simulink model "aeb_sim"  (R2023b)
settings: Solver=ode3  StartTime=0.0  StopTime=t_end  FixedStep=Ts  RelTol=1e-3
values from neighbouring files (symbols this model uses):
  a_cmd_max = 9    [aeb_parameter.m]
  AEB_enable = true    [aeb_parameter.m]
  ax_emergency = 0.90*g    (= 8.829)    [aeb_parameter.m]
  ax_moderate = 0.70*g    (= 6.867)    [aeb_parameter.m]
  ax_partial = 0.45*g    (= 4.4145)    [aeb_parameter.m]
  bias_TTC = 0.05    [aeb_parameter.m]
  CdA = 0.65    [aeb_parameter.m]
  Crr = 0.020    (= 0.02)    [aeb_parameter.m]
  ego_v0 = 27.77    [aeb_parameter.m]
  ego_x0 = 0.0    (= 0)    [aeb_parameter.m]
  eps_v = 0.05    [aeb_parameter.m]
  g = 9.81    [aeb_parameter.m]
  jerk_lim = 20    [aeb_parameter.m]
  m = 2000    [aeb_parameter.m]
  mu = struct('dry',mu_dry,'wet',mu_wet,'ice',mu_ice).(mu_case)    [aeb_parameter.m]
  R_safe = 2.0    (= 2)    [aeb_parameter.m]
  rho_air = 1.2    [aeb_parameter.m]
  tau_brk = 0.08    [aeb_parameter.m]
  tgt_a = -4    [aeb_parameter.m]
  tgt_v0 = 20.83    [aeb_parameter.m]
  tgt_x0 = 45    [aeb_parameter.m]
  TTCbrk = 1.8    [aeb_parameter.m]
  TTCfull = 1.2    [aeb_parameter.m]
  TTClow = 2.6    [aeb_parameter.m]
settings Model: Creator=PRATIK  LastModifiedBy=PRATIK
settings DataIOCC: SaveState=on
settings OptimizationCC: UseDivisionForNetSlopeComputation=on

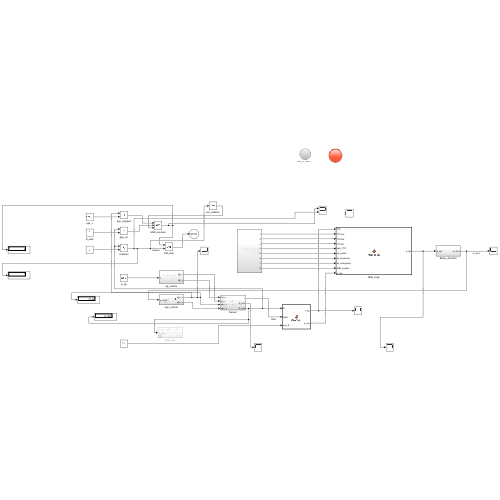
[thumbnail: Simulink's stored preview of the top-level diagram]
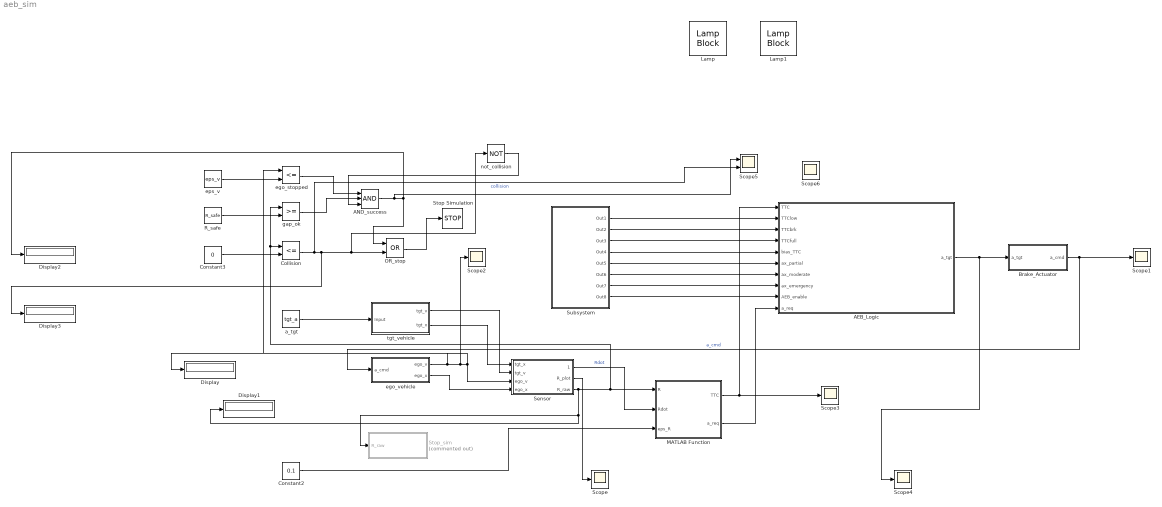
== system aeb_sim ==
  AEB_Logic : MATLAB Function  TreatAsAtomicUnit=on
  AND_success : Logic  Inputs=3  AllPortsSameDT=off  OutDataTypeStr=boolean
  Brake_Actuator : Subsystem
  Collision : RelationalOperator  Operator=<=  OutDataTypeStr=boolean  RndMeth=Simplest  InputSameDT=off
  Constant2 : Constant  Value=0.1
  Constant3 : Constant  Value=0
  Display{,1..3} (4 alike) : Display
  Lamp : LampBlock  LabelPosition=Bottom
  Lamp1 : LampBlock  LabelPosition=Hide
  MATLAB Function : MATLAB Function  TreatAsAtomicUnit=on
  OR_stop : Logic  Operator=OR  AllPortsSameDT=off  OutDataTypeStr=boolean
  R_safe : Constant  Value=R_safe
  Scope{,1..4,6} (6 alike) : Scope
  Scope5 : Scope  NumInputPorts=2
  Sensor : Subsystem
  Stop Simulation : Stop
  Stop_sim : Subsystem  Commented=on
  Subsystem : Subsystem
  a_tgt : Constant  Value=tgt_a
  ego_stopped : RelationalOperator  Operator=<=  OutDataTypeStr=boolean  RndMeth=Simplest  InputSameDT=off
  ego_vehicle : Subsystem
  eps_v : Constant  Value=eps_v
  gap_ok : RelationalOperator  OutDataTypeStr=boolean  RndMeth=Simplest  InputSameDT=off
  not_collision : Logic  Operator=NOT  AllPortsSameDT=off  OutDataTypeStr=boolean
  tgt_vehicle : Subsystem
  wires:
  tgt_vehicle/2(tgt_x) -> Sensor/1(tgt_x)
  tgt_vehicle/1(tgt_v) -> Sensor/2(tgt_v)
  ego_vehicle/1(ego_v) -> Display/1, Scope2/1, Sensor/3(ego_v), ego_stopped/1
  ego_vehicle/2(ego_x) -> Sensor/4(ego_x)
  Constant2/1 -> MATLAB Function/3(eps_R)
  Sensor/1(1) -> MATLAB Function/2(Rdot)  "Rdot"
  Sensor/2(R_plot) -> Scope/1
  MATLAB Function/2(a_req) -> AEB_Logic/10(a_req)
  MATLAB Function/1(TTC) -> Scope3/1, AEB_Logic/1(TTC)
  Subsystem/1(Out1) -> AEB_Logic/2(TTClow)
  Subsystem/2(Out2) -> AEB_Logic/3(TTCbrk)
  Subsystem/3(Out3) -> AEB_Logic/4(TTCfull)
  Subsystem/4(Out4) -> AEB_Logic/5(bias_TTC)
  Subsystem/5(Out5) -> AEB_Logic/6(ax_partial)
  Subsystem/6(Out6) -> AEB_Logic/7(ax_moderate)
  Subsystem/7(Out7) -> AEB_Logic/8(ax_emergency)
  Subsystem/8(Out8) -> AEB_Logic/9(AEB_enable)
  AEB_Logic/1(a_tgt) -> Scope4/1, Brake_Actuator/1(a_tgt)
  Sensor/3(R_raw) -> Stop_sim/1(R_raw), Display1/1, Collision/1, gap_ok/1, MATLAB Function/1(R)
  a_tgt/1 -> tgt_vehicle/1(Input)
  Brake_Actuator/1(a_cmd) -> Scope1/1, ego_vehicle/1(a_cmd)  "a_cmd"
  eps_v/1 -> ego_stopped/2
  R_safe/1 -> gap_ok/2
  Constant3/1 -> Collision/2
  ego_stopped/1 -> AND_success/1
  gap_ok/1 -> AND_success/2
  Collision/1 -> Scope5/2, Display3/1, not_collision/1, OR_stop/2  "collision"
  AND_success/1 -> Scope5/1, OR_stop/1, Display2/1
  OR_stop/1 -> Stop Simulation/1
  not_collision/1 -> AND_success/3

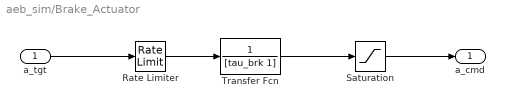
== system aeb_sim/Brake_Actuator ==
  a_tgt : Inport
  Rate Limiter : RateLimiter  RisingSlewLimit=jerk_lim  FallingSlewLimit=-jerk_lim  SampleTimeMode=inherited
  Saturation : Saturate  UpperLimit=min(a_cmd_max, mu*g)  LowerLimit=0
  Transfer Fcn : TransferFcn  Denominator=[tau_brk 1]
  a_cmd : Outport
  wires:
  a_tgt/1 -> Rate Limiter/1
  Rate Limiter/1 -> Transfer Fcn/1
  Transfer Fcn/1 -> Saturation/1
  Saturation/1 -> a_cmd/1

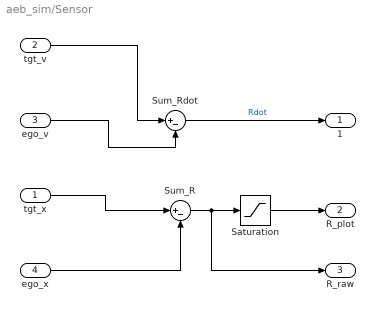
== system aeb_sim/Sensor ==
  tgt_x : Inport
  tgt_v : Inport  Port=2
  ego_v : Inport  Port=3
  ego_x : Inport  Port=4
  Saturation : Saturate  UpperLimit=inf  LowerLimit=0
  Sum_R : Sum  Inputs=|+-
  Sum_Rdot : Sum  Inputs=|+-
  1 : Outport
  R_plot : Outport  Port=2
  R_raw : Outport  Port=3
  wires:
  tgt_x/1 -> Sum_R/1
  ego_x/1 -> Sum_R/2
  ego_v/1 -> Sum_Rdot/2
  tgt_v/1 -> Sum_Rdot/1
  Sum_R/1 -> R_raw/1, Saturation/1
  Saturation/1 -> R_plot/1
  Sum_Rdot/1 -> 1/1  "Rdot"

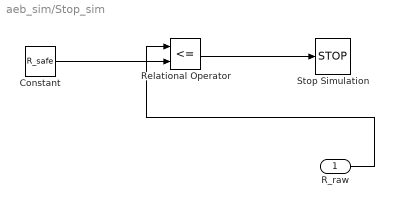
== system aeb_sim/Stop_sim ==
  R_raw : Inport
  Constant : Constant  Value=R_safe
  Relational Operator : RelationalOperator  Operator=<=  OutDataTypeStr=boolean  RndMeth=Simplest  InputSameDT=off
  Stop Simulation : Stop
  wires:
  Relational Operator/1 -> Stop Simulation/1
  R_raw/1 -> Relational Operator/1
  Constant/1 -> Relational Operator/2

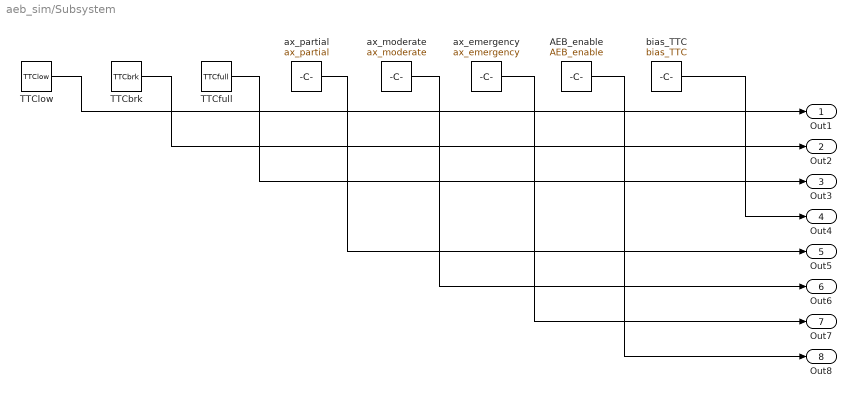
== system aeb_sim/Subsystem ==
  AEB_enable : Constant  Value=AEB_enable
  TTCbrk : Constant  Value=TTCbrk
  TTCfull : Constant  Value=TTCfull
  TTClow : Constant  Value=TTClow
  ax_emergency : Constant  Value=ax_emergency
  ax_moderate : Constant  Value=ax_moderate
  ax_partial : Constant  Value=ax_partial
  bias_TTC : Constant  Value=bias_TTC
  Out1 : Outport
  Out2 : Outport  Port=2
  Out3 : Outport  Port=3
  Out4 : Outport  Port=4
  Out5 : Outport  Port=5
  Out6 : Outport  Port=6
  Out7 : Outport  Port=7
  Out8 : Outport  Port=8
  wires:
  TTClow/1 -> Out1/1
  TTCbrk/1 -> Out2/1
  TTCfull/1 -> Out3/1
  ax_partial/1 -> Out5/1
  bias_TTC/1 -> Out4/1
  AEB_enable/1 -> Out8/1
  ax_moderate/1 -> Out6/1
  ax_emergency/1 -> Out7/1

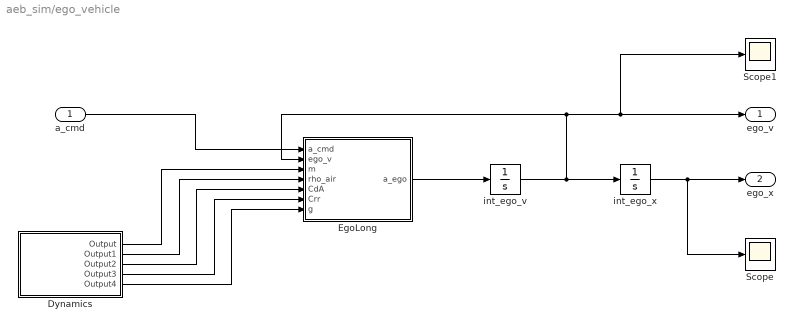
== system aeb_sim/ego_vehicle ==
  a_cmd : Inport
  Dynamics : Subsystem
  EgoLong : MATLAB Function  TreatAsAtomicUnit=on
  Scope : Scope
  Scope1 : Scope
  int_ego_v : Integrator  InitialCondition=ego_v0  LimitOutput=on  LowerSaturationLimit=0
  int_ego_x : Integrator  InitialCondition=ego_x0
  ego_v : Outport
  ego_x : Outport  Port=2
  wires:
  int_ego_v/1 -> ego_v/1, Scope1/1, EgoLong/2(ego_v), int_ego_x/1
  int_ego_x/1 -> Scope/1, ego_x/1
  a_cmd/1 -> EgoLong/1(a_cmd)
  Dynamics/1(Output) -> EgoLong/3(m)
  Dynamics/2(Output1) -> EgoLong/4(rho_air)
  Dynamics/3(Output2) -> EgoLong/5(CdA)
  Dynamics/4(Output3) -> EgoLong/6(Crr)
  Dynamics/5(Output4) -> EgoLong/7(g)
  EgoLong/1(a_ego) -> int_ego_v/1

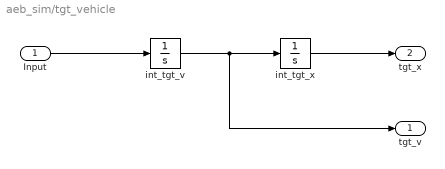
== system aeb_sim/tgt_vehicle ==
  Input : Inport
  int_tgt_v : Integrator  InitialCondition=tgt_v0  LimitOutput=on  LowerSaturationLimit=0
  int_tgt_x : Integrator  InitialCondition=tgt_x0
  tgt_v : Outport
  tgt_x : Outport  Port=2
  wires:
  Input/1 -> int_tgt_v/1
  int_tgt_v/1 -> tgt_v/1, int_tgt_x/1
  int_tgt_x/1 -> tgt_x/1

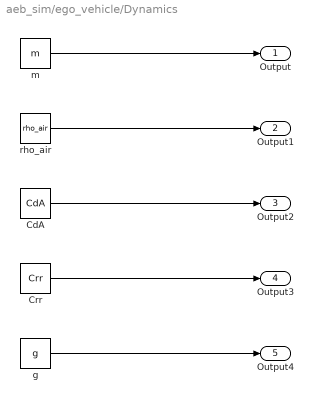
== system aeb_sim/ego_vehicle/Dynamics ==
  CdA : Constant  Value=CdA
  Crr : Constant  Value=Crr
  g : Constant  Value=g
  m : Constant  Value=m
  rho_air : Constant  Value=rho_air
  Output : Outport
  Output1 : Outport  Port=2
  Output2 : Outport  Port=3
  Output3 : Outport  Port=4
  Output4 : Outport  Port=5
  wires:
  m/1 -> Output/1
  rho_air/1 -> Output1/1
  CdA/1 -> Output2/1
  Crr/1 -> Output3/1
  g/1 -> Output4/1

== matlab function aeb_sim/AEB_Logic ==
  data: TTC input; a_tgt output; TTClow input; TTCbrk input; TTCfull input; bias_TTC input; ax_partial input; ax_moderate input; ax_emergency input; AEB_enable input; a_req input
function a_tgt = AEB_Logic(TTC,TTClow,TTCbrk,TTCfull,bias_TTC, ...
                           ax_partial,ax_moderate,ax_emergency, ...
                           AEB_enable,a_req)
% Outputs brake demand a_tgt [m/s^2]
if ~AEB_enable
    a_tgt = 0; 
    return;
end

% Base demand from TTC thresholds (3 levels)
if ~isfinite(TTC)
    base = 0;                         % not closing
elseif TTC <= (TTCfull - bias_TTC)
    base = ax_emergency;
elseif TTC <= TTCbrk
    base = ax_moderate;
elseif TTC <= TTClow
    base = ax_partial;
else
    base = 0;
end

% Ensure enough braking but never exceed emergency
a_tgt = max(base, min(ax_emergency, a_req));
a_tgt = max(0, a_tgt);                % safety clamp
end

== matlab function aeb_sim/MATLAB Function ==
  data: TTC output; R input; Rdot input; eps_R input; a_req output
function [TTC, a_req] = RiskCalc(R, Rdot, eps_R)            % Inputs:  R [m], Rdot [m/s], eps_R ~ 0.1 (numerical guard), % Outputs: TTC [s], a_req [m/s^2]

TTC   = inf;                                                % defaults to avoid "unset" warnings
a_req = 0;
                                                        
R = max(R, eps_R);                                          % 1) guard tiny range


if Rdot < 0                                                 % 2) TTC: only when closing
    den = min(Rdot, -1e-6);                                 % keep negative & away from 0
    TTC = -R / den;                                         % positive seconds
end

   
if Rdot < 0                                                 % 3) required constant decel to avoid impact
    a_req = (Rdot.^2) / (2*R);
else
    a_req = 0;
end
end

== matlab function aeb_sim/ego_vehicle/EgoLong ==
  data: a_cmd input; a_ego output; ego_v input; m input; rho_air input; CdA input; Crr input; g input
function a_ego = EgoLong(a_cmd, ego_v, m, rho_air, CdA, Crr, g)
F_brk  = m*a_cmd;
F_drag = 0.5*rho_air*CdA*ego_v*abs(ego_v);
F_roll = m*g*Crr;
a_ego  = -(F_brk + F_drag + F_roll)/m;   % applied (negative) accel
end
